simulink model "cv9_sim"  (R2019b)
settings: Solver=FixedStepAuto  StartTime=0.0  StopTime=Tsim  FixedStep=Ts  RelTol=1e-3
values from neighbouring files (symbols this model uses):
  D = 1.5    [cv9.m]
  F_uro = feedback(F_oro,1)    [cv9.m]
  I = 1    [cv9.m]
  K = 2    [cv9.m]
  N = 5    [cv9.m]
  P = 2    [cv9.m]
  T = 5    [cv9.m]
settings Model: Creator=Martin Dodek  LastModifiedBy=Martin Dodek

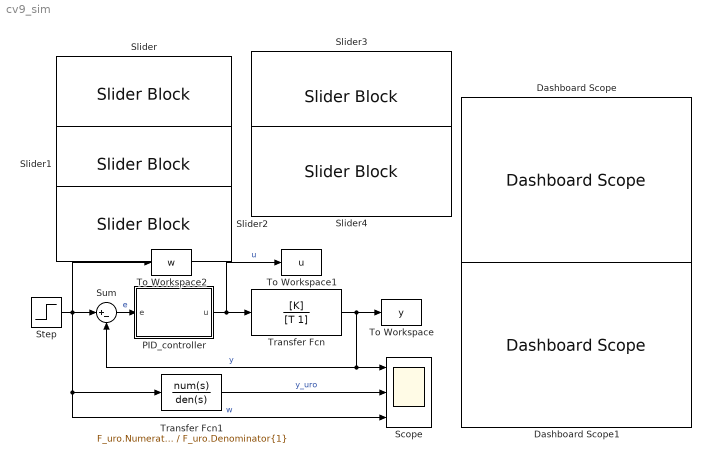
== system cv9_sim ==
  Dashboard Scope : DashboardScope
  Dashboard Scope1 : DashboardScope
  PID_controller : Subsystem
  Scope : Scope  NumInputPorts=3
  Slider : SliderBlock  ScaleMax=10
  Slider1 : SliderBlock  ScaleMax=10
  Slider2 : SliderBlock  ScaleMax=5
  Slider3 : SliderBlock  ScaleMin=0.1  ScaleMax=10
  Slider4 : SliderBlock  ScaleMax=20
  Step : Step  Time=2  SampleTime=0
  Sum : Sum  Inputs=|+-
  To Workspace : ToWorkspace  VariableName=y  SampleTime=-1
  To Workspace1 : ToWorkspace  VariableName=u  SampleTime=-1
  To Workspace2 : ToWorkspace  VariableName=w  SampleTime=-1
  Transfer Fcn : TransferFcn  Numerator=[K]  Denominator=[T 1]
  Transfer Fcn1 : TransferFcn  Numerator=F_uro.Numerator{1}  Denominator=F_uro.Denominator{1}
  wires:
  PID_controller/1(u) -> To Workspace1/1, Transfer Fcn/1  "u"
  Sum/1 -> PID_controller/1(e)  "e"
  Step/1 -> To Workspace2/1, Transfer Fcn1/1, Scope/3, Sum/1  "w"
  Transfer Fcn/1 -> To Workspace/1, Scope/1, Sum/2  "y"
  Transfer Fcn1/1 -> Scope/2  "y_uro"

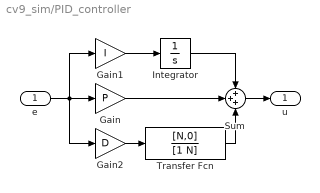
== system cv9_sim/PID_controller ==
  e : Inport
  Gain : Gain  Gain=P
  Gain1 : Gain  Gain=I
  Gain2 : Gain  Gain=D
  Integrator : Integrator
  Sum : Sum  Inputs=+++
  Transfer Fcn : TransferFcn  Numerator=[N,0]  Denominator=[1 N]
  u : Outport
  wires:
  Sum/1 -> u/1
  Gain/1 -> Sum/2
  Gain1/1 -> Integrator/1
  e/1 -> Gain2/1, Gain1/1, Gain/1
  Gain2/1 -> Transfer Fcn/1
  Transfer Fcn/1 -> Sum/3
  Integrator/1 -> Sum/1
